simulink model "flanger"  (R2024a)
settings: Solver=VariableStepAuto  StartTime=0.0  StopTime=20  RelTol=1e-3
libraries: hdlsllib x2
settings Model: Creator=EAGLEAORUS  LastModifiedBy=fermata

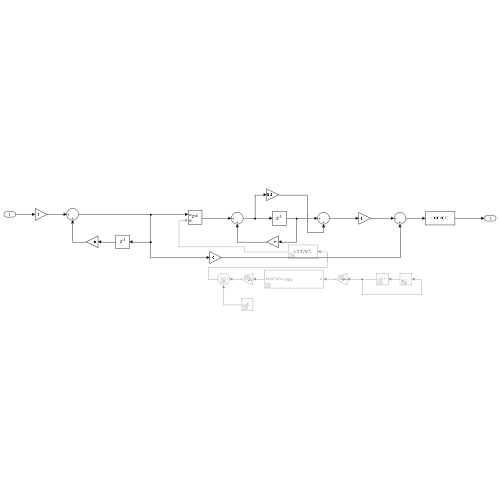
[thumbnail: Simulink's stored preview of the top-level diagram]
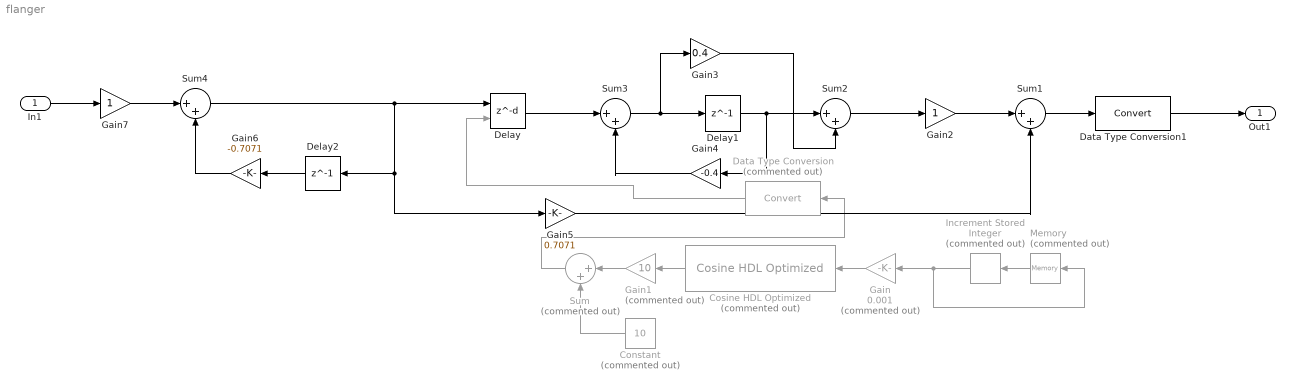
== system flanger ==
  In1 : Inport  OutDataTypeStr=int16
  Constant : Constant  Commented=on  Value=10
  Cosine HDL Optimized : hdlsllib/Lookup Tables/Cosine HDL Optimized  Commented=on  OutputFormula=sin(2*pi*u)  NumDataPoints=1024  TableDataTypeStr=fixdt(0,16,15)  SimulateLUTROMDelay=off
  Data Type Conversion : DataTypeConversion  Commented=on  RndMeth=Round  SaturateOnIntegerOverflow=off
  Data Type Conversion1 : DataTypeConversion  SaturateOnIntegerOverflow=off  RndMeth=Floor
  Delay : Delay  DelayLengthSource=Input port  DelayLength=1  DelayLengthUpperLimit=1024  InitialCondition=0  UseCircularBuffer=on
      settings: InputPortMap=u0,p1
  Delay1 : Delay  DelayLength=1  DelayLengthUpperLimit=1024  InitialCondition=0  UseCircularBuffer=on
  Delay2 : Delay  DelayLength=1  InitialCondition=0
  Gain : Gain  Commented=on  Gain=0.001
  Gain1 : Gain  Commented=on  Gain=10
  Gain2 : Gain
  Gain3 : Gain  Gain=0.4
  Gain4 : Gain  Gain=-0.4  OutDataTypeStr=Inherit: Inherit via back propagation
  Gain5 : Gain  Gain=0.7071
  Gain6 : Gain  Gain=-0.7071  OutDataTypeStr=Inherit: Inherit via back propagation
  Gain7 : Gain
  Increment Stored Integer : hdlsllib/Math Operations/Increment Stored Integer  Commented=on
  Memory : Memory  Commented=on  InheritSampleTime=on
  Sum : Sum  Commented=on  Inputs=|++
  Sum{1..4} (4 alike) : Sum  Inputs=|++
  Out1 : Outport  OutDataTypeStr=int16
  wires:
  Cosine HDL Optimized/1 -> Gain1/1
  Memory/1 -> Increment Stored Integer/1
  Increment Stored Integer/1 -> Memory/1, Gain/1
  Gain/1 -> Cosine HDL Optimized/1
  Gain1/1 -> Sum/1
  Sum/1 -> Data Type Conversion/1
  Delay1/1 -> Sum2/1, Gain4/1
  Sum3/1 -> Gain3/1, Delay1/1
  Gain4/1 -> Sum3/2
  Gain3/1 -> Sum2/2
  Gain2/1 -> Sum1/1
  Sum1/1 -> Data Type Conversion1/1
  Constant/1 -> Sum/2
  Data Type Conversion/1 -> Delay/2
  Gain5/1 -> Sum1/2
  In1/1 -> Gain7/1
  Sum4/1 -> Delay2/1, Gain5/1, Delay/1
  Delay2/1 -> Gain6/1
  Gain6/1 -> Sum4/2
  Sum2/1 -> Gain2/1
  Delay/1 -> Sum3/1
  Data Type Conversion1/1 -> Out1/1
  Gain7/1 -> Sum4/1
